simulink model "model"  (Simulink 10.1)
settings: Solver=FixedStepAuto  StartTime=0.0  StopTime=30.0  FixedStep=0.01  RelTol=1e-3  EnableMultiTasking=on
model workspace (MAT data in the model file):
  Kd = 10
  Ki = 1
  Kp : num (value not decoded)
values from neighbouring files (symbols this model uses):
  g = 9.81    [fcn1.m]
undefined symbols (not defined in the file or in its folder): a1, a2, a3, a4, a5, b1, b2, b3, Kf, Km, m
settings Model: Creator=Felipe Vargas  LastModifiedBy=nikhil
settings DataIOCC: LimitDataPoints=on
settings DebuggingCC: UnderspecifiedInitializationDetection=Simplified  MergeDetectMultiDrivingBlocksExec=error
settings GRTTargetCC: CombineOutputUpdateFcns=on  GRTInterface=off

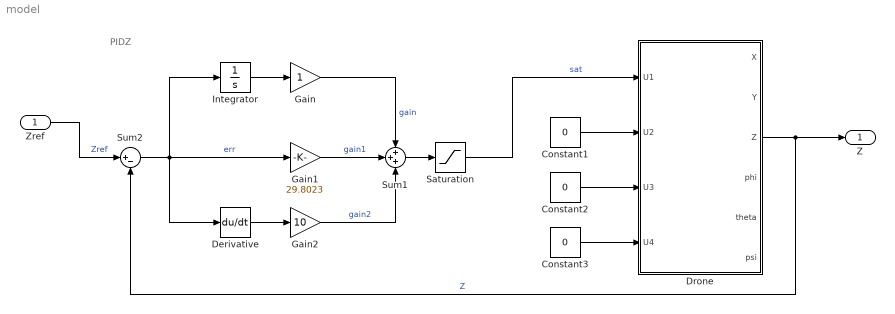
== system model ==
  note: PIDZ
  Zref : Inport
  Constant1 : Constant  Value=0
  Constant2 : Constant  Value=0
  Constant3 : Constant  Value=0
  Derivative : Derivative
  Drone : Subsystem
  Gain : Gain
  Gain1 : Gain  Gain=29.8023
  Gain2 : Gain  Gain=10
  Integrator : Integrator
  Saturation : Saturate  UpperLimit=15  LowerLimit=-15
  Sum1 : Sum  Inputs=+++
  Sum2 : Sum  Inputs=|+-
  Z : Outport
  wires:
  Drone/3(Z) -> Z/1, Sum2/2  "Z"
  Zref/1 -> Sum2/1  "Zref"
  Constant1/1 -> Drone/2(U2)
  Constant2/1 -> Drone/3(U3)
  Constant3/1 -> Drone/4(U4)
  Saturation/1 -> Drone/1(U1)  "sat"
  Gain/1 -> Sum1/1  "gain"
  Sum1/1 -> Saturation/1
  Gain1/1 -> Sum1/2  "gain1"
  Derivative/1 -> Gain2/1
  Sum2/1 -> Derivative/1, Gain1/1, Integrator/1  "err"
  Gain2/1 -> Sum1/3  "gain2"
  Integrator/1 -> Gain/1

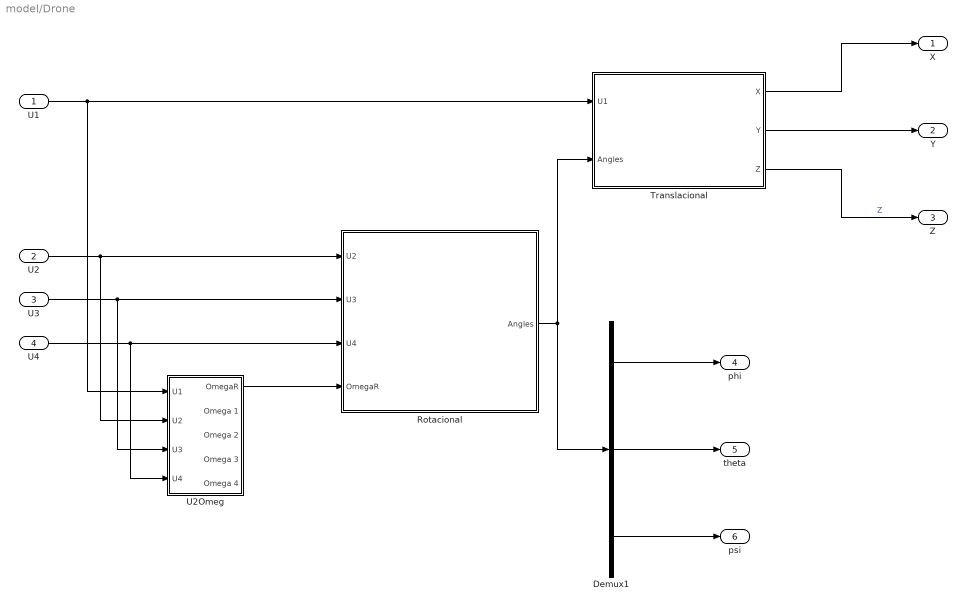
== system model/Drone ==
  U1 : Inport
  U2 : Inport  Port=2
  U3 : Inport  Port=3
  U4 : Inport  Port=4
  Demux1 : Demux  Outputs=3
  Rotacional : Subsystem
  Translacional : Subsystem
  U2Omeg : Subsystem
  X : Outport
  Y : Outport  Port=2
  Z : Outport  Port=3
  phi : Outport  Port=4
  theta : Outport  Port=5
  "psi " : Outport  Port=6
  wires:
  Rotacional/1(Angles) -> Translacional/2(Angles), Demux1/1
  Demux1/1 -> phi/1
  Demux1/2 -> theta/1
  Demux1/3 -> "psi "/1
  Translacional/1(X) -> X/1
  Translacional/3(Z) -> Z/1  "Z"
  Translacional/2(Y) -> Y/1
  U2/1 -> U2Omeg/2("U2 "), Rotacional/1(U2)
  U1/1 -> Translacional/1(U1), U2Omeg/1("U1 ")
  U4/1 -> U2Omeg/4("U4 "), Rotacional/3(U4)
  U3/1 -> U2Omeg/3("U3 "), Rotacional/2(U3)
  U2Omeg/1(OmegaR) -> Rotacional/4(OmegaR)

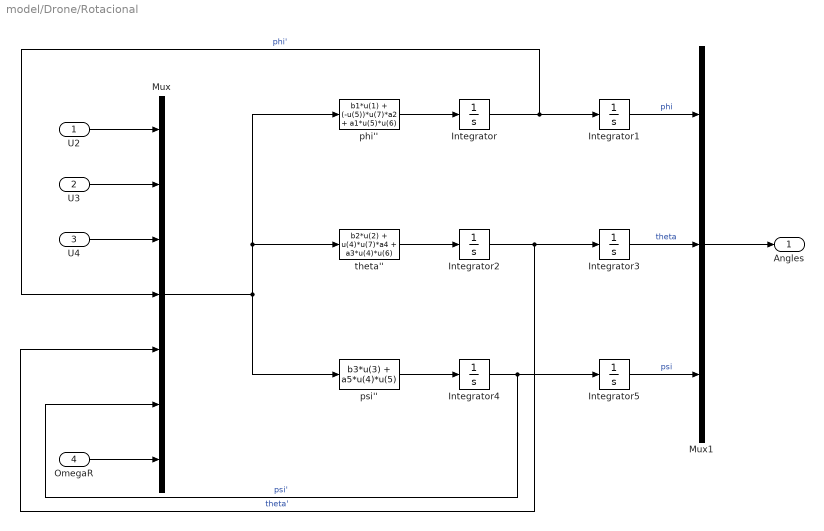
== system model/Drone/Rotacional ==
  U2 : Inport
  U3 : Inport  Port=2
  U4 : Inport  Port=3
  OmegaR : Inport  Port=4
  Integrator{,1..5} (6 alike) : Integrator
  Mux : Mux  Inputs=7
  Mux1 : Mux  Inputs=3
  phi'' : Fcn  Expr=b1*u(1) + (-u(5))*u(7)*a2 + a1*u(5)*u(6)
  psi'' : Fcn  Expr=b3*u(3) + a5*u(4)*u(5)
  theta'' : Fcn  Expr=b2*u(2) + u(4)*u(7)*a4 + a3*u(4)*u(6)
  Angles : Outport
  wires:
  U2/1 -> Mux/1
  U3/1 -> Mux/2
  U4/1 -> Mux/3
  phi''/1 -> Integrator/1
  Integrator/1 -> Mux/4, Integrator1/1  "phi'"
  Mux/1 -> psi''/1, theta''/1, phi''/1
  theta''/1 -> Integrator2/1
  Integrator2/1 -> Mux/5, Integrator3/1  "theta'"
  psi''/1 -> Integrator4/1
  Integrator4/1 -> Mux/6, Integrator5/1  "psi'"
  Integrator1/1 -> Mux1/1  "phi"
  Integrator3/1 -> Mux1/2  "theta"
  Mux1/1 -> Angles/1
  Integrator5/1 -> Mux1/3  "psi"
  OmegaR/1 -> Mux/7

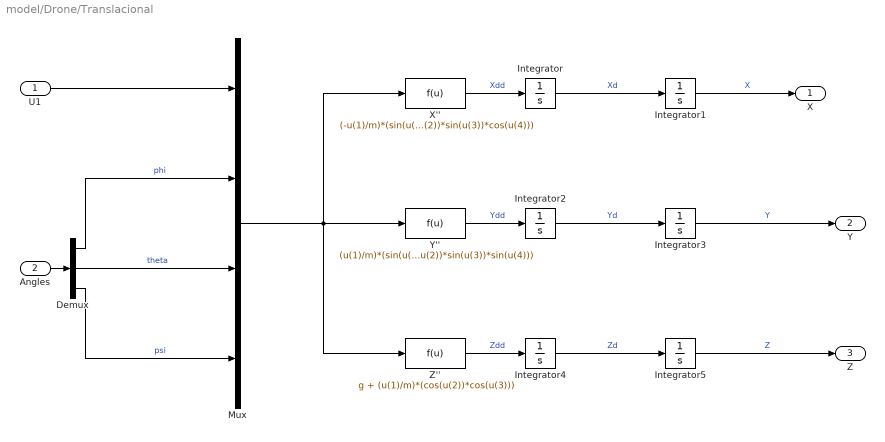
== system model/Drone/Translacional ==
  U1 : Inport
  Angles : Inport  Port=2
  Demux : Demux  Outputs=3
  Integrator{,1..5} (6 alike) : Integrator
  Mux : Mux
  X'' : Fcn  Expr=(-u(1)/m)*(sin(u(2))*sin(u(4)) + cos(u(2))*sin(u(3))*cos(u(4)))
  Y'' : Fcn  Expr=(u(1)/m)*(sin(u(2))*cos(u(4)) - cos(u(2))*sin(u(3))*sin(u(4)))
  Z'' : Fcn  Expr=g + (u(1)/m)*(cos(u(2))*cos(u(3)))
  X : Outport
  Y : Outport  Port=2
  Z : Outport  Port=3
  wires:
  X''/1 -> Integrator/1  "Xdd"
  Integrator/1 -> Integrator1/1  "Xd"
  Angles/1 -> Demux/1
  Mux/1 -> Z''/1, Y''/1, X''/1
  U1/1 -> Mux/1
  Demux/1 -> Mux/2  "phi"
  Demux/2 -> Mux/3  "theta"
  Demux/3 -> Mux/4  "psi"
  Y''/1 -> Integrator2/1  "Ydd"
  Integrator2/1 -> Integrator3/1  "Yd"
  Integrator3/1 -> Y/1  "Y"
  Z''/1 -> Integrator4/1  "Zdd"
  Integrator4/1 -> Integrator5/1  "Zd"
  Integrator5/1 -> Z/1  "Z"
  Integrator1/1 -> X/1  "X"

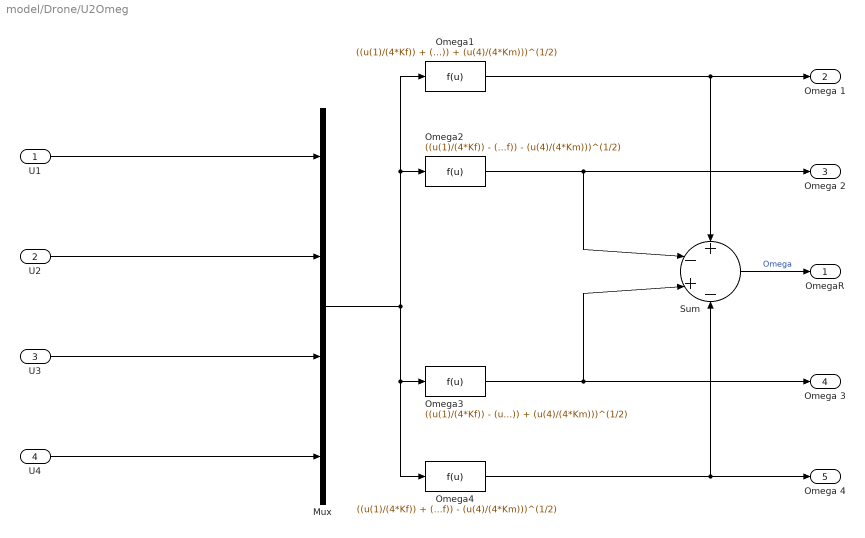
== system model/Drone/U2Omeg ==
  "U1 " : Inport
  "U2 " : Inport  Port=2
  "U3 " : Inport  Port=3
  "U4 " : Inport  Port=4
  Mux : Mux
  Omega1 : Fcn  Expr=((u(1)/(4*Kf)) + (u(3)/(2*Kf)) + (u(4)/(4*Km)))^(1/2)
  Omega2 : Fcn  Expr=((u(1)/(4*Kf)) - (u(2)/(2*Kf)) - (u(4)/(4*Km)))^(1/2)
  Omega3 : Fcn  Expr=((u(1)/(4*Kf)) - (u(3)/(2*Kf)) + (u(4)/(4*Km)))^(1/2)
  Omega4 : Fcn  Expr=((u(1)/(4*Kf)) + (u(2)/(2*Kf)) - (u(4)/(4*Km)))^(1/2)
  Sum : Sum  Inputs=+-+-
  OmegaR : Outport
  Omega 1 : Outport  Port=2
  Omega 2 : Outport  Port=3
  Omega 3 : Outport  Port=4
  Omega 4 : Outport  Port=5
  wires:
  Omega2/1 -> Sum/2, Omega 2/1
  Omega1/1 -> Sum/1, Omega 1/1
  Omega3/1 -> Sum/3, Omega 3/1
  Mux/1 -> Omega2/1, Omega1/1, Omega4/1, Omega3/1
  Omega4/1 -> Omega 4/1, Sum/4
  "U4 "/1 -> Mux/4
  "U3 "/1 -> Mux/3
  "U2 "/1 -> Mux/2
  "U1 "/1 -> Mux/1
  Sum/1 -> OmegaR/1  "Omega"
